simulink model "system_dyninv_1st_order_distrej2"  (R2018b)
settings: Solver=ode8  StartTime=0.0  StopTime=10  FixedStep=0.01  RelTol=1e-3
values from neighbouring files (symbols this model uses):
  A = -4    [dyninv_1st_order_dist.m]    (also in dyninv_1st_order_distrej.m)
  B = 0.5    [dyninv_1st_order_dist.m]    (also in dyninv_1st_order_distrej.m)
  C = 1    [dyninv_1st_order_dist.m]    (also in dyninv_1st_order_distrej.m)
  CA = C*A    (= -4)    [dyninv_1st_order_dist.m]    (also in dyninv_1st_order_distrej.m)
  fc = sqrt(fi)    [dyninv_1st_order_distrej.m]
  invCB = inv(C*B)    [dyninv_1st_order_dist.m]    (also in dyninv_1st_order_distrej.m)
  Kb = 4    [dyninv_1st_order_distrej.m]
settings Model: Creator=suvo.ganguli  LastModifiedBy=suvo.ganguli

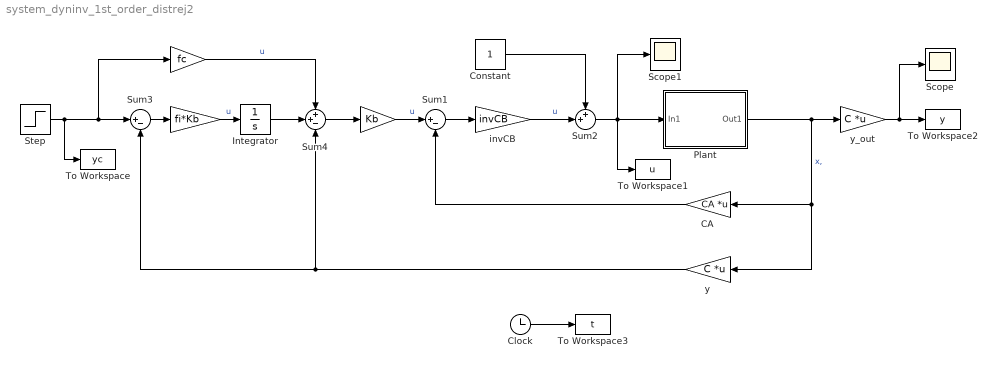
== system system_dyninv_1st_order_distrej2 ==
  " " : Gain  Gain=fi*Kb
  "  " : Gain  Gain=fc
  "   " : Gain  Gain=Kb
  CA : Gain  Gain=CA  Multiplication=Matrix(K*u)
  Clock : Clock
  Constant : Constant
  Integrator : Integrator
  Plant : Subsystem
  Scope : Scope
  Scope1 : Scope
  Step : Step  Time=5  SampleTime=0
  Sum1 : Sum  Inputs=|+-
  Sum2 : Sum  Inputs=++|
  Sum3 : Sum  Inputs=|+-
  Sum4 : Sum  Inputs=++-
  To Workspace : ToWorkspace  VariableName=yc  SampleTime=-1
  To Workspace1 : ToWorkspace  VariableName=u  SampleTime=-1
  To Workspace2 : ToWorkspace  VariableName=y  SampleTime=-1
  To Workspace3 : ToWorkspace  VariableName=t  SampleTime=-1
  invCB : Gain  Gain=invCB
  y : Gain  Gain=C  Multiplication=Matrix(K*u)
  y_out : Gain  Gain=C  Multiplication=Matrix(K*u)
  wires:
  Plant/1(Out1) -> y_out/1, y/1, CA/1  "x,"
  y/1 -> Sum4/3, Sum3/2
  CA/1 -> Sum1/2
  y_out/1 -> To Workspace2/1, Scope/1
  Sum1/1 -> invCB/1
  Clock/1 -> To Workspace3/1
  invCB/1 -> Sum2/2  "u"
  Sum2/1 -> To Workspace1/1, Scope1/1, Plant/1(In1)
  Constant/1 -> Sum2/1
  "   "/1 -> Sum1/1  "u"
  Sum4/1 -> "   "/1
  Integrator/1 -> Sum4/2
  " "/1 -> Integrator/1  "u"
  Sum3/1 -> " "/1
  "  "/1 -> Sum4/1  "u"
  Step/1 -> To Workspace/1, "  "/1, Sum3/1

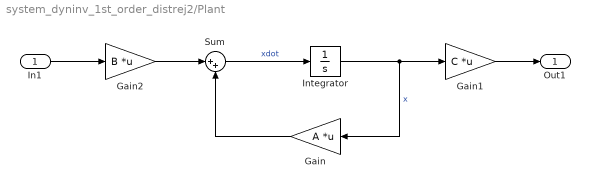
== system system_dyninv_1st_order_distrej2/Plant ==
  In1 : Inport
  Gain : Gain  Gain=A  Multiplication=Matrix(K*u)
  Gain1 : Gain  Gain=C  Multiplication=Matrix(K*u)
  Gain2 : Gain  Gain=B  Multiplication=Matrix(K*u)
  Integrator : Integrator
  Sum : Sum  Inputs=|++
  Out1 : Outport
  wires:
  Integrator/1 -> Gain1/1, Gain/1  "x"
  Sum/1 -> Integrator/1  "xdot"
  Gain/1 -> Sum/2
  In1/1 -> Gain2/1
  Gain2/1 -> Sum/1
  Gain1/1 -> Out1/1
